simulink model "majorPonepointO"  (R2023a)
settings: Solver=VariableStepAuto  StartTime=0.0  StopTime=80.0  RelTol=1e-3
libraries: arduinolib x1
settings Model: Creator=rahul  LastModifiedBy=rahul

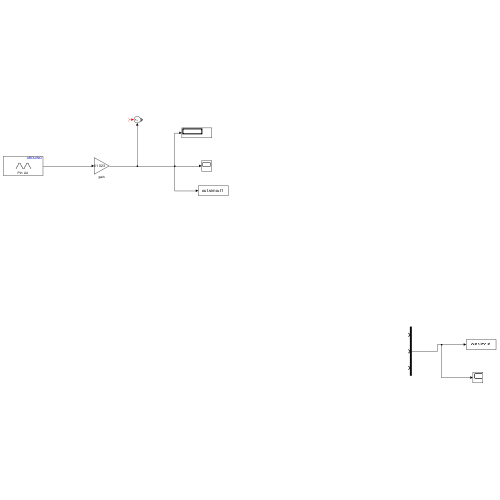
[thumbnail: Simulink's stored preview of the top-level diagram]
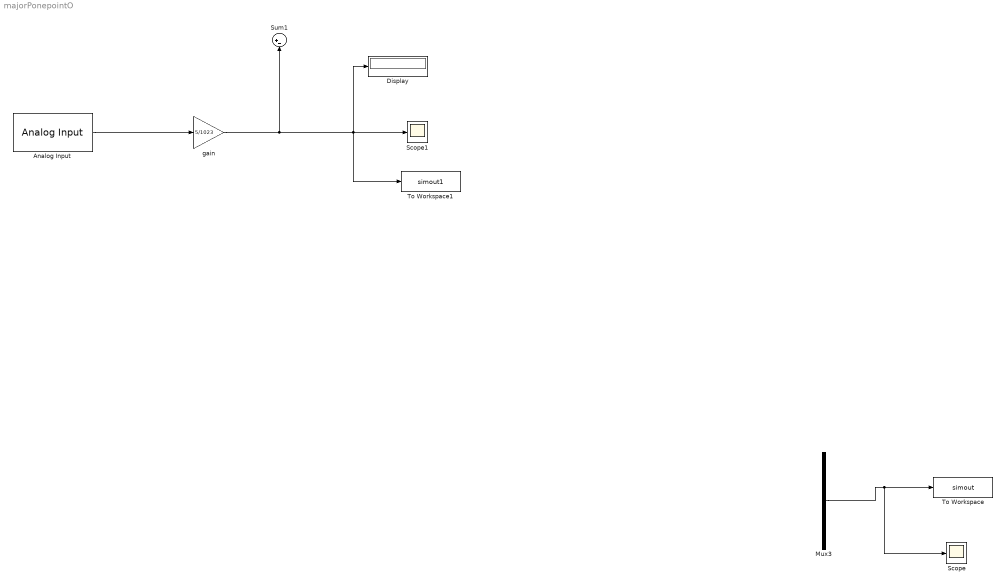
== system majorPonepointO ==
  Analog Input : arduinolib/Analog Input  pinNumber=4  ReadResultsOnly=off  ConversionTriggerSource=Software  ExternalTriggerType=uint32( 0 )  OutputDataType=uint16  EnableConversionCompleteNotify=off  EnableOuputStatus=off  SampleTime=-1  blockPlatform=arduino
  Display : Display
  Mux3 : Mux  Inputs=3
  Scope : Scope
  Scope1 : Scope
  Sum1 : Sum  Inputs=|+-
  To Workspace : ToWorkspace  VariableName=simout  SaveFormat=Timeseries  SampleTime=-1
  To Workspace1 : ToWorkspace  VariableName=simout1  SaveFormat=Timeseries  SampleTime=-1
  gain : Gain  Gain=5/1023
  wires:
  Analog Input/1 -> gain/1
  Mux3/1 -> Scope/1, To Workspace/1
  gain/1 -> Sum1/2, To Workspace1/1, Display/1, Scope1/1
  ? -> Sum1/1
